simulink model "FlipFlopSimo"  (R2019b)
settings: Solver=VariableStepAuto  StartTime=0.0  StopTime=10.0  RelTol=1e-3
undefined symbols (not defined in the file or in its folder): sigbuilder_block
libraries: simulink_extras x1
settings Model: Creator=Simo  LastModifiedBy=utente
settings SolverCC: AlgebraicLoopSolver=LineSearch

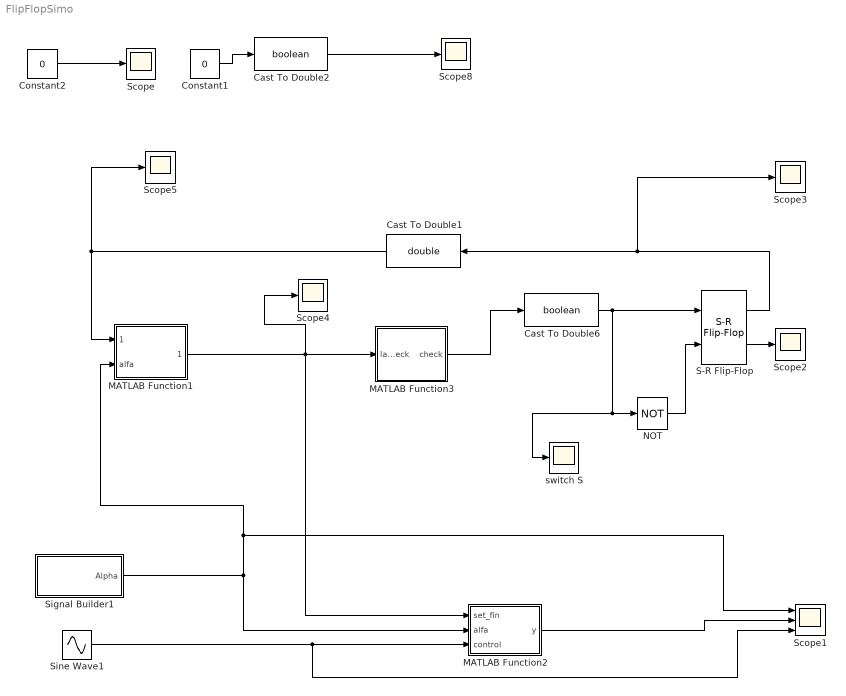
== system FlipFlopSimo ==
  Cast To Double1 : DataTypeConversion  OutDataTypeStr=double
  Cast To Double2 : DataTypeConversion  OutDataTypeStr=boolean
  Cast To Double6 : DataTypeConversion  OutDataTypeStr=boolean
  Constant1 : Constant  Value=0
  Constant2 : Constant  Value=0
  MATLAB Function1 : MATLAB Function  TreatAsAtomicUnit=on
  MATLAB Function2 : MATLAB Function  TreatAsAtomicUnit=on
  MATLAB Function3 : MATLAB Function  TreatAsAtomicUnit=on
  NOT : Logic  Operator=NOT  IconShape=distinctive  AllPortsSameDT=off  OutDataTypeStr=boolean
  S-R Flip-Flop : simulink_extras/Flip Flops/S-R Flip-Flop  initial_condition=0
  Scope{,2..5,8} (6 alike) : Scope
  Scope1 : Scope  NumInputPorts=3
  Signal Builder1 : Subsystem  Tag=STV Subsys  LoadFcn=sigbuilder_block('load');  StartFcn=sigbuilder_block('start');  StopFcn=sigbuilder_block('stop');  ClipboardFcn=sigbuilder_block('clipboard');  mask(Sigbuilder block){tuvar=[0:10]}
      mask help: Simulink:masks:SigbuilderBlock_MD
      mask init:
      | if ~strcmp(get_param(bdroot(gcbh),'SimulationStatus'),'stopped') tuvar = sigbuilder_block('maskInit'); end
      settings: CopyFcn=sigbuilder_block('copy');  DeleteFcn=sigbuilder_block('delete');  ModelCloseFcn=sigbuilder_block('modelClose');  PreSaveFcn=sigbuilder_block('preSave');  PauseFcn=sigbuilder_block('pause');  ContinueFcn=sigbuilder_block('continue');  NameChangeFcn=sigbuilder_block('namechange');  OpenFcn=sigbuilder_block('open',[153.75 63 594.75 258 ]);  CloseFcn=sigbuilder_block('close');
      mask Display: plot(0, 0, 100, 100,[2, 2, 32, 32, 2], [68, 8, 8, 68, 68],[32, 2], [38, 38], [32, 19, 2],[53, 60, 44], [32, 17, 17, 2],[16, 16, 31, 31]);txt = getActiveGroup(gcbh);text(2, 100, txt,'verticalAlignment', 'top');
  Sine Wave1 : Sin  SampleTime=0
  switch S : Scope
  wires:
  Signal Builder1/1(Alpha) -> MATLAB Function2/2(alfa), Scope1/1, MATLAB Function1/2(alfa)
  Sine Wave1/1 -> Scope1/3, MATLAB Function2/3(control)
  MATLAB Function2/1(y) -> Scope1/2
  S-R Flip-Flop/2 -> Scope2/1
  Constant1/1 -> Cast To Double2/1
  Cast To Double2/1 -> Scope8/1
  S-R Flip-Flop/1 -> Cast To Double1/1, Scope3/1
  MATLAB Function1/1(pre_flip) -> MATLAB Function3/1(last_check), MATLAB Function2/1(set_fin), Scope4/1
  MATLAB Function3/1(check) -> Cast To Double6/1
  Cast To Double6/1 -> S-R Flip-Flop/1, NOT/1, switch S/1
  Constant2/1 -> Scope/1
  Cast To Double1/1 -> MATLAB Function1/1(set_value), Scope5/1
  NOT/1 -> S-R Flip-Flop/2

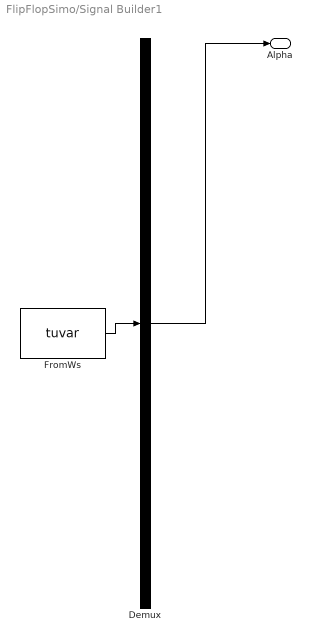
== system FlipFlopSimo/Signal Builder1 ==
  Demux : Demux  Tag=STV Demux  Outputs=1
  FromWs : FromWorkspace  Tag=STV FromWs  VariableName=tuvar  SampleTime=0
      SigBuilderData=|
      | common.afterFinalStr = 'Extrapolate'
      | common.sampleTime = 0
      | dataSet.timeRange = [0 10]
      | dataSet.name = 'Group 1'
      | sbobj.Groups.Name = 'Group 1'
      | sbobj.Groups.Signals.Name = 'Alpha'
      | sbobj.Groups.Signals.XData = [0 2 4 5 6 10]
      | sbobj.Groups.Signals.YData = [8 0 0 4 5 8.2]
  Alpha : Outport  Tag=STV Outport
  wires:
  Demux/1 -> Alpha/1
  FromWs/1 -> Demux/1

== matlab function FlipFlopSimo/MATLAB Function1 ==
  data: set_value input; alfa input; pre_flip output
function pre_flip = fcn(set_value,alfa)
u=0;
    if(alfa==0)
        if(set_value==0)
            u=1;
        end
        if(set_value==1)
            u=2;
        end
    else
        u=0;
    end




pre_flip=u;


    %if (alfa>0.001&&set_value==0)
        %if (set_value==0&&set_value==0)
        %pre_flip=1;
        %else
        %pre_flip=0;
     %   end
      %  if (alfa==0.001&&set_value==1)
       % u=2;
       % pre_flip=2;
        %else
        %pre_flip=0;
        %end
   %else
   % pre_flip=0;
   % end
end

== matlab function FlipFlopSimo/MATLAB Function2 ==
  data: set_fin input; alfa input; y output; control input
function y = fcn(set_fin,alfa,control)
z=0;
   if (-5<=alfa<=5&&set_fin==2)
         z=control;
   end
 y=z;  
end

== matlab function FlipFlopSimo/MATLAB Function3 ==
  data: last_check input; check output
function check = fcn(last_check)
k=0;    
if (last_check==0||last_check==2)
    k=0;   
   % check=u;
end
if(last_check==1)
        k=1;
        %check=u;
end
    check=k;
end
